simulink subsystem "SENSORS"  (R2025b)
settings: Solver=VariableStepAuto  StartTime=0.0  StopTime=10.0  RelTol=1e-3
model mask{gyrUpdateFreq=0, gyrMeasLim=0, magUpdateFreq=0, magMeasLim=0, magNoisePerChannel=0, magNoiseSeeds=0, strUpdateFreq=0, gnssUpdateFreq=0, gnssHorzAcc=0, gnssVertAcc=0, gnssVelAcc=0}
  mask prompts: gyrUpdateFreq "Update frequency [Hz]"; gyrMeasLim "Measurable angular velocity limits [rads-1]"; magUpdateFreq "Update frequency [Hz]"; magMeasLim "Measurable magnetic field per channel [nT]"; magNoisePerChannel "Noise (3 sigma) [nT]"; magNoiseSeeds "Noise seeds"; strUpdateFreq "Update frequency [Hz]"; gnssUpdateFreq "Update frequency [Hz]"; gnssHorzAcc "Horizontal accuracy [m]"; gnssVertAcc "Vertical accuracy [m]"; gnssVelAcc "Velocity accuracy [ms-1]"
libraries: simulink_extras x3, aerolibtransform2 x1, sensorgpslib x1, sharedutil x1, aerolibutil x1, aerolibnav x1
settings Model: Creator=antoniohernandez-rodiciomateos  LastModifiedBy=antoniohernandez-rodiciomateos

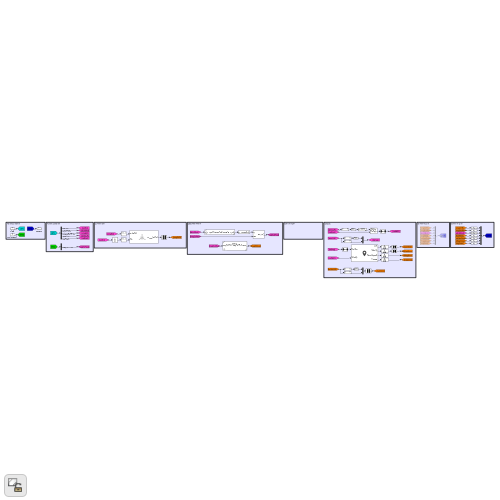
[thumbnail: Simulink's stored preview of the top-level diagram]
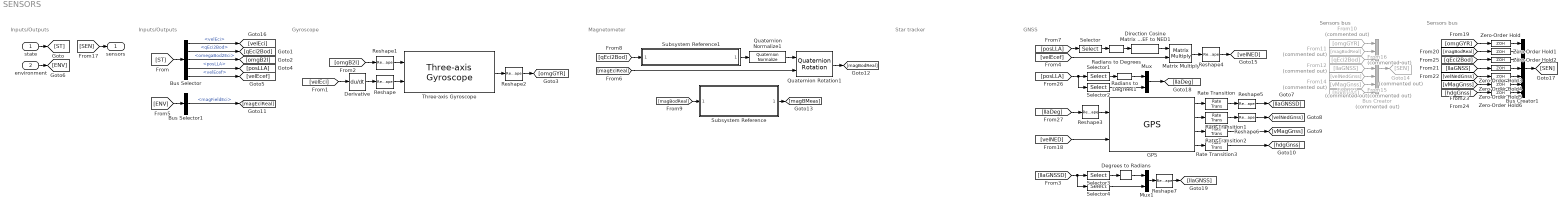
== system SENSORS ==
  note: Inputs/Outputs
  note: Inputs/Outputs
  note: Gyroscope
  note: Magnetometer
  note: Star tracker
  note: GNSS
  note: Sensors bus
  note: Sensors bus
  state : Inport  OutDataTypeStr=Bus: state_bus
  environment : Inport  Port=2
  Bus Creator : BusCreator  Commented=on  Inputs=7  OutDataTypeStr=Bus: sensors_bus  NonVirtualBus=on
      settings: InheritFromInputs=off
  Bus Creator1 : BusCreator  Inputs=7  OutDataTypeStr=Bus: sensors_bus  NonVirtualBus=on
      settings: InheritFromInputs=off
  Bus Selector : BusSelector  OutputSignals=velEci,qEci2Bod,omegaBod2Eci,posLLA,velEcef
  Bus Selector1 : BusSelector  OutputSignals=magFieldEci
  Degrees to Radians : simulink_extras/Transformations/Degrees to Radians
  Derivative : Derivative
  Direction Cosine Matrix ECEF to NED1 : aerolibtransform2/Direction Cosine Matrix ECEF to NED
  From10 : From  Commented=on  GotoTag=omgGYR
  From11 : From  Commented=on  GotoTag=magBodReal
  From12 : From  Commented=on  GotoTag=llaGNSS
  From13 : From  Commented=on  GotoTag=velNedGnss
  From14 : From  Commented=on  GotoTag=vMagGnss
  From15 : From  Commented=on  GotoTag=hdgGnss
  From16 : From  Commented=on  GotoTag=qEci2Bod
  GPS : sensorgpslib/GPS  DispRefFrame=NED  PositionInputFormat=Geodetic  ReferenceLocation=[ 0, 0, 0 ]  HorizontalPositionAccuracy=gnssHorzAcc  VerticalPositionAccuracy=gnssVertAcc  VelocityAccuracy=gnssVelAcc  DecayFactor=0.999  SeedDouble=67  SimulateUsing=Interpreted execution
      settings: LibrarySourceBlock=mspsensorlib/GPS
  Goto14 : Goto  Commented=on  GotoTag=SEN
  Matrix Multiply : Product  Multiplication=Matrix(*)
  Mux : Mux  Inputs=2
  Mux1 : Mux  Inputs=2
  Quaternion Normalize1 : sharedutil/Quaternion Normalize  aMode=aMode
  Quaternion Rotation1 : aerolibutil/Quaternion Rotation
  Radians to Degrees : simulink_extras/Transformations/Radians to Degrees
  Radians to Degrees1 : simulink_extras/Transformations/Radians to Degrees
  Rate Transition{,1..3} (4 alike) : RateTransition  OutPortSampleTime=1 / gnssUpdateFreq
  Reshape : Reshape
  Reshape1 : Reshape
  Reshape{2,5..7} (4 alike) : Reshape  OutputDimensionality=Column vector (2-D)
  Reshape3 : Reshape  OutputDimensionality=Row vector (2-D)
  Reshape4 : Reshape  OutputDimensionality=Row vector (2-D)
  Selector : Selector  InputPortWidth=3  IndexOptions=Index vector (dialog)  Indices=[1:2]  OutputSizes=1
  Selector1 : Selector  InputPortWidth=3  IndexOptions=Index vector (dialog)  Indices=[1:2]  OutputSizes=1
  Selector2 : Selector  InputPortWidth=3  IndexOptions=Index vector (dialog)  Indices=[3]  OutputSizes=1
  Selector3 : Selector  InputPortWidth=3  IndexOptions=Index vector (dialog)  Indices=[1:2]  OutputSizes=1
  Selector4 : Selector  InputPortWidth=3  IndexOptions=Index vector (dialog)  Indices=[3]  OutputSizes=1
  Subsystem Reference : Subsystem  ReferencedSubsystem=MAG  magUpdateFreq=magUpdateFreq  magMeasLim=magMeasLim  magNoisePerChannel=magNoisePerChannel  magNoiseSeed=magNoiseSeeds
  Subsystem Reference1 : Subsystem  ReferencedSubsystem=quatConventionConverter  conversion=q4 to q0
  Three-axis Gyroscope : aerolibnav/Three-axis Gyroscope  dtype_g=on  w_g=190  z_g=0.707  g_sf_cc=[1 0 0; 0 1 0; 0 0 1]  g_bias=[0 0 0]  g_sen=[0 0 0]  g_Ts=1 / gyrUpdateFreq  g_rand=on  g_seeds=[23093 23094 23095]  g_pow=[0.0001 0.0001 0.0001]  g_sat="[-inf  -inf  -inf  inf inf inf]"
  Zero-Order Hold{,1..6} (7 alike) : ZeroOrderHold  SampleTime=0.05
  sensors : Outport  OutDataTypeStr=Bus: sensors_bus
  wires:
  state/1 -> [ST]
  [ST] -> Bus Selector/1
  Bus Selector/1 -> [velEci]  "<velEci>"
  Bus Selector/2 -> [qEci2Bod]  "<qEci2Bod>"
  Bus Selector/3 -> [omgB2I]  "<omegaBod2Eci>"
  Bus Selector/4 -> [posLLA]  "<posLLA>"
  Bus Selector/5 -> [velEcef]  "<velEcef>"
  Reshape3/1 -> GPS/1
  [llaDeg] -> Reshape3/1
  [velEcef] -> Matrix Multiply/2
  Direction Cosine Matrix ECEF to NED1/1 -> Matrix Multiply/1
  Matrix Multiply/1 -> Reshape4/1
  GPS/1 -> Rate Transition/1
  GPS/2 -> Rate Transition1/1
  GPS/3 -> Rate Transition2/1
  GPS/4 -> Rate Transition3/1
  environment/1 -> [ENV]
  [ENV] -> Bus Selector1/1
  Bus Selector1/1 -> [magEciReal]  "<magFieldEci>"
  Quaternion Normalize1/1 -> Quaternion Rotation1/1
  [qEci2Bod] -> Subsystem Reference1/1
  Quaternion Rotation1/1 -> [magBodReal]
  [magEciReal] -> Quaternion Rotation1/2
  Subsystem Reference1/1 -> Quaternion Normalize1/1
  Reshape1/1 -> Three-axis Gyroscope/1
  Reshape/1 -> Three-axis Gyroscope/2
  [omgB2I] -> Reshape1/1
  [velEci] -> Derivative/1
  Derivative/1 -> Reshape/1
  Three-axis Gyroscope/1 -> Reshape2/1
  Reshape2/1 -> [omgGYR]
  From10/1 -> Bus Creator/1
  From11/1 -> Bus Creator/2
  From16/1 -> Bus Creator/3
  From12/1 -> Bus Creator/4
  From13/1 -> Bus Creator/5
  From14/1 -> Bus Creator/6
  From15/1 -> Bus Creator/7
  Bus Creator/1 -> Goto14/1
  [SEN] -> sensors/1
  Rate Transition/1 -> Reshape5/1
  Reshape5/1 -> [llaGNSSD]
  Rate Transition1/1 -> Reshape6/1
  Reshape6/1 -> [velNedGnss]
  Rate Transition2/1 -> [vMagGnss]
  Rate Transition3/1 -> [hdgGnss]
  [posLLA] -> Selector/1
  Selector/1 -> Radians to Degrees/1
  Radians to Degrees/1 -> Direction Cosine Matrix ECEF to NED1/1
  Reshape4/1 -> [velNED]
  [velNED] -> GPS/2
  Bus Creator1/1 -> [SEN]
  [omgGYR] -> Zero-Order Hold/1
  Zero-Order Hold/1 -> Bus Creator1/1
  Zero-Order Hold1/1 -> Bus Creator1/2
  [magBodReal] -> Zero-Order Hold1/1
  Zero-Order Hold2/1 -> Bus Creator1/3
  [qEci2Bod] -> Zero-Order Hold2/1
  [llaGNSS] -> Zero-Order Hold3/1
  Zero-Order Hold4/1 -> Bus Creator1/5
  Zero-Order Hold3/1 -> Bus Creator1/4
  Zero-Order Hold5/1 -> Bus Creator1/6
  [vMagGnss] -> Zero-Order Hold5/1
  [velNedGnss] -> Zero-Order Hold4/1
  Zero-Order Hold6/1 -> Bus Creator1/7
  [hdgGnss] -> Zero-Order Hold6/1
  [posLLA] -> Selector1/1, Selector2/1
  Selector1/1 -> Radians to Degrees1/1
  Selector2/1 -> Mux/2
  Radians to Degrees1/1 -> Mux/1
  Mux/1 -> [llaDeg]
  Degrees to Radians/1 -> Mux1/1
  Selector3/1 -> Degrees to Radians/1
  Selector4/1 -> Mux1/2
  [llaGNSSD] -> Selector3/1, Selector4/1
  Mux1/1 -> Reshape7/1
  Reshape7/1 -> [llaGNSS]
  Subsystem Reference/1 -> [magBMeas]
  [magBodReal] -> Subsystem Reference/1
